simulink model "Emulate_Prescan_2019a"  (R2019a)
settings: Solver=FixedStepDiscrete  StartTime=0.0  StopTime=30  FixedStep=1  RelTol=1e-3
libraries: robotlib x2
settings Model: Creator=jinglei  LastModifiedBy=adeye
settings OptimizationCC: EnhancedBackFolding=on  PassReuseOutputArgsAs=Individual arguments  MaxStackSize=64  OptimizeBlockOrder=speed  DifferentSizesBufferReuse=on  OptimizationCustomize=off
settings DebuggingCC: ParameterTunabilityLossMsg=error  SFUnexpectedBacktrackingDiag=warning  SFNoUnconditionalDefaultTransitionDiag=warning
settings HardwareCC: ProdBitPerPointer=32  ProdBitPerSizeT=32  ProdBitPerPtrDiffT=32  ProdLargestAtomicFloat=None  ProdIntDivRoundTo=Undefined  ProdEndianess=Unspecified  ProdWordSize=32  ProdHWDeviceType=Generic->Unspecified (assume 32-bit Generic)  UseEmbeddedCoderFeatures=off
settings SFSimCC: MATLABDynamicMemAlloc=off
settings RTWCC: SystemTargetFile=ert.tlc  HardwareBoard=Robot Operating System (ROS)  TLCOptions="-aInlineSetEventsForThisBaseRateFcn=TLC_FALSE -aSuppressMultiTaskScheduler=TLC_FALSE  -aRateBasedStepFcn=0"  TemplateMakefile=ert_default_tmf  GenerateReport=on  Toolchain=Catkin  BuildConfiguration=Debug  IncludeHyperlinkInReport=on  LaunchReport=on  TargetLang=C++  GenerateTraceInfo=on  GenerateTraceReport=on  GenerateTraceReportSl=on  GenerateTraceReportSf=on  GenerateTraceReportEml=on
settings CodeAppCC: ForceParamTrailComments=on  IgnoreCustomStorageClasses=off  OperatorAnnotations=on  SimulinkDataObjDesc=on  SFDataObjDesc=on  InsertBlockDesc=on  EnableCustomComments=on
settings ERTTargetCC: SupportNonInlinedSFcns=on

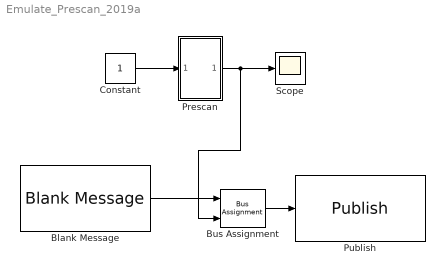
== system Emulate_Prescan_2019a ==
  Blank Message : robotlib/Blank Message  messageClass=Message  entityType=std_msgs/UInt16  messageType=std_msgs/UInt16  SampleTime=inf
      settings: SourceProductBaseCode=RO
  Bus Assignment : BusAssignment  AssignedSignals=Data
  Constant : Constant  OutDataTypeStr=uint16
  Prescan : Subsystem
  Publish : robotlib/Publish  topicSource=Specify your own  topic=/counter  messageType=std_msgs/UInt16  messageQueueLength=1
      settings: SourceProductBaseCode=RO
  Scope : Scope
  wires:
  Constant/1 -> Prescan/1(In1)
  Prescan/1(Out1) -> Bus Assignment/2, Scope/1
  Blank Message/1 -> Bus Assignment/1
  Bus Assignment/1 -> Publish/1

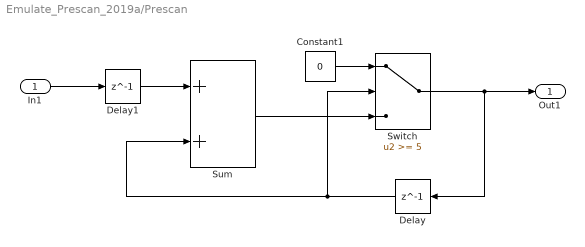
== system Emulate_Prescan_2019a/Prescan ==
  In1 : Inport
  Constant1 : Constant  Value=0
  Delay : Delay  DelayLength=1
  Delay1 : Delay  DelayLength=1
  Sum : Sum
  Switch : Switch  Threshold=5
  Out1 : Outport
  wires:
  Delay/1 -> Switch/2, Sum/2
  Constant1/1 -> Switch/1
  Delay1/1 -> Sum/1
  In1/1 -> Delay1/1
  Switch/1 -> Out1/1, Delay/1
  Sum/1 -> Switch/3
